simulink subsystem "thermal_model_stage_2"  (R2023a)
settings: Solver=VariableStepAuto  StartTime=0.0  StopTime=10.0  RelTol=1e-3
undefined symbols (not defined in the file or in its folder): coolant_initial_pressure, coolant_initial_temperature, coolant_tube_D, tcp_port_diameter, tcp_time_constant, tcv_orifice_diameter, tcv_time_constant
libraries: fl_lib x24, nesl_utility x21, SimscapeFluids_lib x4
settings Model: Creator=stefan.notter  LastModifiedBy=stefan.notter
settings OptimizationCC: ReuseModelBlockBuffer=off

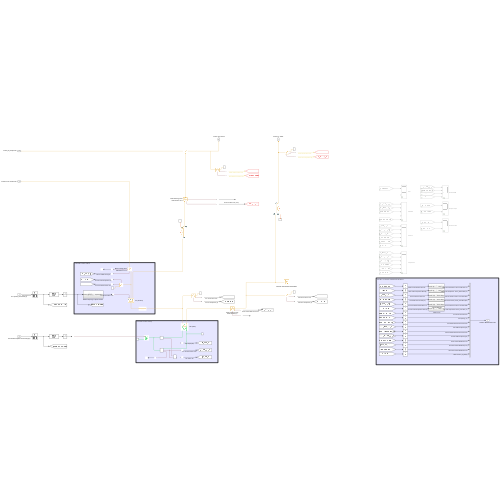
[thumbnail: Simulink's stored preview of the top-level diagram]
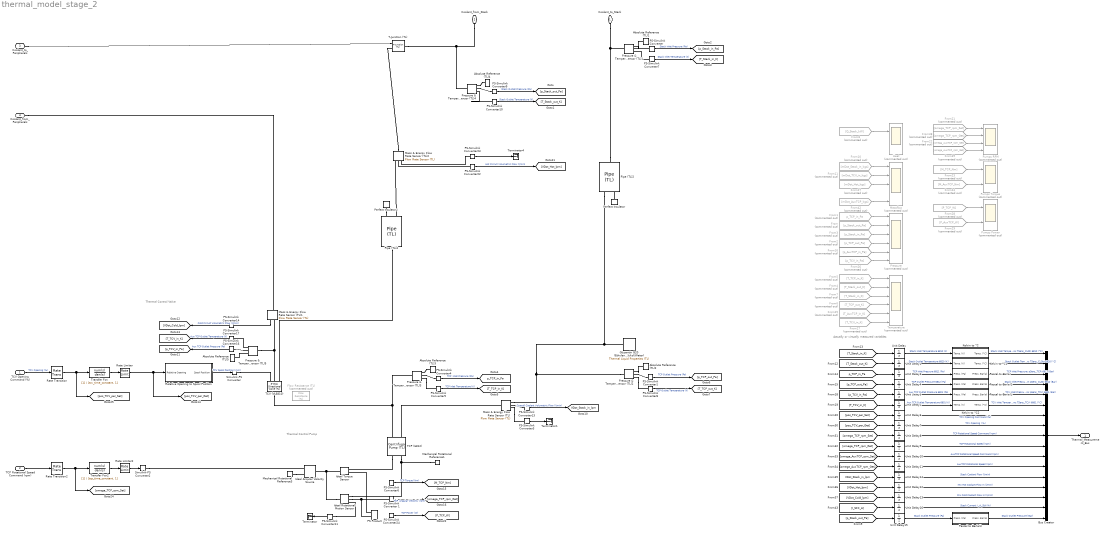
== system thermal_model_stage_2 ==
  note: Thermal Control Valve
  note: Actually or virtually measured variables
  note: Thermal Control Pump
  TCV Opening Command (%) : Inport
  TCP Rotational Speed Command (rpm) : Inport  Port=2
  Absolute Reference (TL){1..5} (5 alike) : fl_lib/Thermal Liquid/Elements/Absolute Reference (TL)
  Bus Creator : BusCreator  Inputs=17
  Flow Resistance (TL) : fl_lib/Thermal Liquid/Elements/Flow Resistance (TL)  Commented=on  delta_p_nominal=0.05 bar  mdot_nominal=1 kg/s  area=pi*tcv_orifice_diameter^2/4 m^2  laminar_fraction=1e-3
  From : From  Commented=on  GotoTag=p_Stack_out_Pa
  From1 : From  Commented=on  GotoTag=p_TCP_in_Pa  TagVisibility=global
  From10 : From  Commented=on  GotoTag=mDot_Stack_in_kgs  TagVisibility=global
  From11 : From  Commented=on  GotoTag=mDot_TCV_in_kgs
  From16 : From  Commented=on  GotoTag=p_AuxTCP_in_Pa
  From17 : From  Commented=on  GotoTag=T_TCV_in_K
  From2 : From  Commented=on  GotoTag=p_TCP_out_Pa
  From21 : From  Commented=on  GotoTag=omega_TCP_rpm_Set
  From22 : From  Commented=on  GotoTag=omega_AuxTCP_rpm_Set
  From23 : From  Commented=on  GotoTag=M_TCP_Nm
  From24 : From  Commented=on  GotoTag=M_AuxTCP_Nm
  From25 : From  Commented=on  GotoTag=T_AuxTCP_in_K
  From26 : From  Commented=on  GotoTag=p_TCV_in_Pa
  From27 : From  Commented=on  GotoTag=mDot_Hot_kgs
  From28 : From  Commented=on  GotoTag=P_TCP_W
  From29 : From  Commented=on  GotoTag=P_AuxTCP_W
  From3 : From  Commented=on  GotoTag=p_Stack_in_Pa
  From38 : From  Commented=on  GotoTag=omega_TCP_rpm_Get
  From39 : From  Commented=on  GotoTag=omega_AuxTCP_rpm_Get
  From4 : From  Commented=on  GotoTag=T_Stack_out_K
  From42 : From  Commented=on  GotoTag=mDot_AuxTCP_kgs
  From5 : From  Commented=on  GotoTag=T_TCP_in_K
  From6 : From  Commented=on  GotoTag=T_TCP_out_K
  From7 : From  Commented=on  GotoTag=T_Stack_in_K
  From8 : From  Commented=on  GotoTag=Q_Stack_kW  TagVisibility=global
  Glysantin G20 (Ethylenglykol/Water) : SimscapeFluids_lib/Thermal Liquid/Utilities/Thermal Liquid Properties (TL)  fluid_list=fluids.thermal_liquid.utilities.enum.thermal_liquid_fluid_list.ethylene_glycol  concentration_param_EG=fluids.thermal_liquid.utilities.enum.thermal_liquid_concentration.volume_fraction  concentration_param_PG=fluids.thermal_liquid.utilities.enum.thermal_liquid_concentration.volume_fraction  c_mass_SW=3.5e-3  c_mass_EG=0.1  c_mass_PG=0.1  c_mass_GL=0.1  c_vol_EG=0.5  c_vol_PG=0.1  beta_const_EG=2.1791 GPa  beta_const_PG=2.1791 GPa  beta_const_GL=2.1791 GPa  p_min_EG=0.01 MPa  p_min_PG=0.01 MPa  p_min_GL=0.01 MPa  p_max_EG=50 MPa  p_max_PG=50 MPa  p_max_GL=50 MPa  p_atm=coolant_initial_pressure MPa  properties_range_check=simscape.enum.assert.action.error
  Heat : Scope  Commented=on  NumInputPorts=2
  Ideal Angular Velocity Source : fl_lib/Mechanical/Mechanical Sources/Ideal Angular Velocity Source
  Ideal Rotational Motion Sensor : fl_lib/Mechanical/Mechanical Sensors/Ideal Rotational Motion Sensor  reference=foundation.enum.MeasurementReference.difference  acceleration_port=false  velocity_port=true  position_port=true  wrap_angle=false  offset=0 rad
  Ideal Torque Sensor : fl_lib/Mechanical/Mechanical Sensors/Ideal Torque Sensor
  Kelvin to °C : Subsystem
  Kelvin to °C1 : Subsystem
  Kelvin to °C2 : Subsystem
  Mass & Energy Flow Rate Sensor (TL) : fl_lib/Thermal Liquid/Sensors/Flow Rate Sensor (TL)  mass_flow_measure=false  volumetric_flow_measure=true  energy_flow_measure=true
      settings: InternalSimscapePortConfiguration="{\"Bottom\":[{\"id\":\"PHI\",\"label\":\"φ\",\"type\":\"output\"}],\"Left\":[{\"id\":\"A\",\"label\":\"A\",\"type\":\"foundation.thermal_liquid.thermal_liquid\"}],\"Right\":[{\"id\":\"B\",\"label\":\"B\",\"type\":\"foundation.thermal_liquid.thermal_liquid\"},{\"id\":\"V\",\"label\":\"V\",\"type\":\"output\"}],\"Top\":[]}"
  Mass & Energy Flow Rate Sensor (TL)1 : fl_lib/Thermal Liquid/Sensors/Flow Rate Sensor (TL)  mass_flow_measure=false  volumetric_flow_measure=true  energy_flow_measure=false
      settings: InternalSimscapePortConfiguration="{\"Bottom\":[],\"Left\":[{\"id\":\"A\",\"label\":\"A\",\"type\":\"foundation.thermal_liquid.thermal_liquid\"}],\"Right\":[{\"id\":\"B\",\"label\":\"B\",\"type\":\"foundation.thermal_liquid.thermal_liquid\"},{\"id\":\"V\",\"label\":\"V\",\"type\":\"output\"}],\"Top\":[]}"
  Mass & Energy Flow Rate Sensor (TL)2 : fl_lib/Thermal Liquid/Sensors/Flow Rate Sensor (TL)  mass_flow_measure=false  volumetric_flow_measure=true  energy_flow_measure=true
      settings: InternalSimscapePortConfiguration="{\"Bottom\":[{\"id\":\"PHI\",\"label\":\"φ\",\"type\":\"output\"}],\"Left\":[{\"id\":\"A\",\"label\":\"A\",\"type\":\"foundation.thermal_liquid.thermal_liquid\"}],\"Right\":[{\"id\":\"B\",\"label\":\"B\",\"type\":\"foundation.thermal_liquid.thermal_liquid\"},{\"id\":\"V\",\"label\":\"V\",\"type\":\"output\"}],\"Top\":[]}"
  Massflow : Scope  Commented=on  NumInputPorts=5
  Mechanical Rotational Reference1 : fl_lib/Mechanical/Rotational Elements/Mechanical Rotational Reference
  Mechanical Rotational Reference3 : fl_lib/Mechanical/Rotational Elements/Mechanical Rotational Reference
  PS Product : fl_lib/Physical Signals/Functions/PS Product
  PS-Simulink Converter{,1,3..5,7..11,16..17,23} (13 alike) : nesl_utility/PS-Simulink Converter  PhysicalDomain=network_engine_domain  SubClassName=ps_output  LeftPortType=input  RightPortType=output  PseudoPeriodic=off  Frequencies=[]  VectorFormat=inherit  Unit=inherit  AffineConversion=off
  PS-Simulink Converter 1 : nesl_utility/PS-Simulink Converter  PhysicalDomain=network_engine_domain  SubClassName=ps_output  LeftPortType=input  RightPortType=output  PseudoPeriodic=off  Frequencies=[]  VectorFormat=1-D array  Unit=rpm  AffineConversion=off
  PS-Simulink Converter13 : nesl_utility/PS-Simulink Converter  PhysicalDomain=network_engine_domain  SubClassName=ps_output  LeftPortType=input  RightPortType=output  PseudoPeriodic=off  Frequencies=[]  VectorFormat=inherit  Unit=l/min  AffineConversion=off
  PS-Simulink Converter14 : nesl_utility/PS-Simulink Converter  PhysicalDomain=network_engine_domain  SubClassName=ps_output  LeftPortType=input  RightPortType=output  PseudoPeriodic=off  Frequencies=[]  VectorFormat=inherit  Unit=l/min  AffineConversion=off
  PS-Simulink Converter22 : nesl_utility/PS-Simulink Converter  PhysicalDomain=network_engine_domain  SubClassName=ps_output  LeftPortType=input  RightPortType=output  PseudoPeriodic=off  Frequencies=[]  VectorFormat=inherit  Unit=l/min  AffineConversion=off
  PS-Simulink Converter24 : nesl_utility/PS-Simulink Converter  PhysicalDomain=network_engine_domain  SubClassName=ps_output  LeftPortType=input  RightPortType=output  PseudoPeriodic=off  Frequencies=[]  VectorFormat=inherit  Unit=W  AffineConversion=off
  PS-Simulink Converter6 : nesl_utility/PS-Simulink Converter  PhysicalDomain=network_engine_domain  SubClassName=ps_output  LeftPortType=input  RightPortType=output  PseudoPeriodic=off  Frequencies=[]  VectorFormat=inherit  Unit=N*m  AffineConversion=off
  Pascal to Bar(a) : Subsystem
  Pascal to Bar(a)1 : Subsystem
  Pascal to Bar(a)2 : Subsystem
  Pascal to Bar(a)3 : Subsystem
  Perfect Insulator : fl_lib/Thermal/Thermal Elements/Perfect Insulator  T_specify=off  T_priority=None  T=293.15 K  T_nominal_specify=off  T_nominal_unit=K  T_nominal_value=1
  Perfect Insulator2 : fl_lib/Thermal/Thermal Elements/Perfect Insulator  T_specify=off  T_priority=None  T=293.15 K  T_nominal_specify=off  T_nominal_unit=K  T_nominal_value=1
  Pipe (TL)2 : fl_lib/Thermal Liquid/Elements/Pipe (TL)  length=0.5 m  area=pi*coolant_tube_D^2/4 m^2  Dh=pi*coolant_tube_D*0.9 m  length_add=1 m  roughness=15e-6 m  Re_lam=2000  Re_tur=4000  shape_factor=64  Nu_lam=3.66  dynamic_compressibility=simscape.enum.onoff.on  inertia=simscape.enum.onoff.off  p0=coolant_initial_pressure MPa  T0=coolant_initial_temperature K  mdot0=0 kg/s
  Pipe (TL)4 : fl_lib/Thermal Liquid/Elements/Pipe (TL)  length=0.5 m  area=pi*coolant_tube_D^2/4 m^2  Dh=pi*coolant_tube_D*0.9 m  length_add=1 m  roughness=15e-6 m  Re_lam=2000  Re_tur=4000  shape_factor=64  Nu_lam=3.66  dynamic_compressibility=simscape.enum.onoff.on  inertia=simscape.enum.onoff.off  p0=coolant_initial_pressure MPa  T0=coolant_initial_temperature K  mdot0=0 kg/s
  Pressure : Scope  Commented=on  NumInputPorts=6
  Pressure & Temperature Sensor (TL){1..5} (5 alike) : fl_lib/Thermal Liquid/Sensors/Pressure & Temperature Sensor (TL)  reference=foundation.enum.MeasurementReference.difference  pressure=true  pressure_spec=foundation.enum.PressureMeasementSpec.Absolute  temperature=true
      settings: InternalSimscapePortConfiguration="{\"Bottom\":[{\"id\":\"T\",\"label\":\"T\",\"type\":\"output\"}],\"Left\":[{\"id\":\"A\",\"label\":\"A\",\"type\":\"foundation.thermal_liquid.thermal_liquid\"}],\"Right\":[{\"id\":\"B\",\"label\":\"B\",\"type\":\"foundation.thermal_liquid.thermal_liquid\"},{\"id\":\"P\",\"label\":\"P\",\"type\":\"output\"}],\"Top\":[]}"
  Pumps Power : Scope  Commented=on  NumInputPorts=2
  Pumps RPM : Scope  Commented=on  NumInputPorts=4
  Pumps Torque : Scope  Commented=on  NumInputPorts=2
  Rate Limiter : RateLimiter  RisingSlewLimit=45  FallingSlewLimit=-45  SampleTimeMode=inherited
  Rate Limiter2 : RateLimiter  RisingSlewLimit=1000  FallingSlewLimit=-1000  SampleTimeMode=inherited
  Rate Transition : RateTransition
  Rate Transition2 : RateTransition
  Relative Opening to Spool Position : Subsystem
  Simulink-PS Converter : nesl_utility/Simulink-PS Converter  PhysicalDomain=network_engine_domain  SubClassName=ps_input  LeftPortType=input  RightPortType=output  PseudoPeriodic=off  Frequencies=[]  NoiseDistribution=none  NoiseParameters=[]  Unit=mm  AffineConversion=off  FilteringAndDerivatives=provide  SimscapeFilterOrder=1  InputFilterTimeConstant=0.001  UdotUserProvided=0
  Simulink-PS Converter2 : nesl_utility/Simulink-PS Converter  PhysicalDomain=network_engine_domain  SubClassName=ps_input  LeftPortType=input  RightPortType=output  PseudoPeriodic=off  Frequencies=[]  NoiseDistribution=none  NoiseParameters=[]  Unit=rpm  AffineConversion=off  FilteringAndDerivatives=provide  SimscapeFilterOrder=1  InputFilterTimeConstant=0.001  UdotUserProvided=0
  T-Junction (TL) : SimscapeFluids_lib/Thermal Liquid/Pipes & Fittings/T-Junction (TL)  area_main=pi*coolant_tube_D^2/4 m^2  area_branch=pi*coolant_tube_D^2/4 m^2  junction_spec=fluids.thermal_liquid.pipes_fittings.enum.TLossCoefficientModel.Crane  k_main_converge=1.12  k_main_diverge=1.12  k_branch_converge=1.12  k_branch_diverge=1.12  radius=0.001 m  Re_c=150  saturation_ratio=0.2  mdot_A_specify=off  mdot_A_priority=High  mdot_A=0 kg/s  mdot_A_nominal_specify=off  mdot_A_nominal_unit=kg/s  mdot_A_nominal_value=1  mdot_B_specify=off  mdot_B_priority=High  mdot_B=0 kg/s  mdot_B_nominal_specify=off  mdot_B_nominal_unit=kg/s  mdot_B_nominal_value=1  mdot_C_specify=off  mdot_C_priority=High  mdot_C=0 kg/s  mdot_C_nominal_specify=off  mdot_C_nominal_unit=kg/s  mdot_C_nominal_value=1
      settings: InternalSimscapePortConfiguration="{\"Bottom\":[{\"id\":\"C\",\"label\":\"C\",\"type\":\"foundation.thermal_liquid.thermal_liquid\"}],\"Left\":[{\"id\":\"A\",\"label\":\"A\",\"type\":\"foundation.thermal_liquid.thermal_liquid\"}],\"Right\":[{\"id\":\"B\",\"label\":\"B\",\"type\":\"foundation.thermal_liquid.thermal_liquid\"}],\"Top\":[]}"
  TCP (6812) : SimscapeFluids_lib/Thermal Liquid/Pumps & Motors/Centrifugal Pump (TL)  pump_parameterization=fluids.thermal_liquid.pumps_motors.enum.CentrifugalPumpParameterization.Table2D  capacity_ref_nominal=6000/60 lpm  head_ref_nominal=|  power_ref_nominal=0.3 kW  head_ref_max=|  capacity_ref_max=12000/60 lpm  omega_ref_analytic=3500 rpm  flow_rate_1D_TLU=[1000, 2000, 3000, 4000, 5000, 6000, 7000, 8000, 9000, 1000] lpm  head_1D_TLU=[50, 47.5, 45, 40, 35, 25] m  power_1D_TLU=[.6, .75, .85, .93, .98, .99] kW  omega_ref_1D=3500 rpm  rho_ref_1D=998.21 kg/m^3  omega_threshold_factor=1e-2  flow_rate_2D_TLU=tcp_capacity_vector_lpm lpm  omega_2D_TLU=tcp_shaft_speed_vector_rpm rpm  head_2D_TLU=tcp_head_table_m m  power_2D_TLU=tcp_brake_power_table_kW kW  rho_ref_2D=tcp_reference_density kg/m^3  diameter_ratio=1  mech_orientation=fluids.thermal_liquid.pumps_motors.enum.CentrifugalPumpMechOrientation.Positive  area=pi/4*tcp_port_diameter^2 m^2
      head_ref_nominal=|
      | 1.2*10^5/(1000*9.81)
      |  m
      head_ref_max=|
      | 1.55*10^5/(1000*9.81)
      |  m
      settings: InternalSimscapePortConfiguration="{\"Bottom\":[],\"Left\":[{\"id\":\"A\",\"label\":\"A\",\"type\":\"foundation.thermal_liquid.thermal_liquid\"},{\"id\":\"B\",\"label\":\"B\",\"type\":\"foundation.thermal_liquid.thermal_liquid\"}],\"Right\":[{\"id\":\"R\",\"label\":\"R\",\"type\":\"foundation.mechanical.rotational.rotational\"},{\"id\":\"C\",\"label\":\"C\",\"type\":\"foundation.mechanical.rotational.rotational\"}],\"Top\":[]}"
  TCV (VL6810) : SimscapeFluids_lib/Thermal Liquid/Valves & Orifices/Directional Control Valves/3-Way Directional Valve (TL)  open_orifices_pos=fluids.thermal_liquid.valves.directional_control_valves.enum.OpenOrifices3Way.PA  open_orifices_neg=fluids.thermal_liquid.valves.directional_control_valves.enum.OpenOrifices3Way.AT  area_spec=fluids.thermal_liquid.valves.directional_control_valves.enum.area_spec.identical  valve_spec=fluids.thermal_liquid.valves.directional_control_valves.enum.ValveSpec.Table1DAreaOpening  del_S_max=5e-3 m  area_max=pi*tcv_orifice_diameter^2/4 m^2  del_S_TLU=tcv_spool_travel_vec m  valve_area_TLU=tcv_orifice_area_vec m^2  del_S_flow_TLU=[0, .002, .004, .007, .017] m  p_diff_TLU=[.3, .5, .7] bar  vol_flow_TLU=1e-3 * [1.7e-05, 2e-05, 2.6e-05; .0035, .0045, .0053; .7, .9, 1.06; 1.96, 2.5, 3; 6, 7.7, 9.13] lpm  mdot_TLU=[1.7e-05, 2e-05, 2.6e-05; .0035, .0045, .0053; .7, .9, 1.06; 1.96, 2.5, 3; 6, 7.7, 9.13] kg/s  T_ref_in=293.15 K  p_ref_in=0.101325 MPa  area_leak=tcv_leakage_area m^2  Cd=0.7  Re_c=12  smoothing_factor=0.01  pressure_recovery=simscape.enum.onoff.off  area=pi*coolant_tube_D^2/4 m^2  S_max_PA=2.5e-3 m  del_S_max_PA=0.005 m  area_max_PA=1e-4 m^2  del_S_TLU_PA=[0, .002, .004, .007, .017] m  valve_area_TLU_PA=[1e-09, 2.0352e-07, 4.0736e-05, .00011438, .00034356] m^2  del_S_flow_TLU_PA=[0, .002, .004, .007, .017] m  p_diff_TLU_PA=[.3, .5, .7] MPa  vol_flow_TLU_PA=1e-3 * [1.7e-05, 2e-05, 2.6e-05; .0035, .0045, .0053; .7, .9, 1.06; 1.96, 2.5, 3; 6, 7.7, 9.13] m^3/s  mdot_TLU_PA=[1.7e-05, 2e-05, 2.6e-05; .0035, .0045, .0053; .7, .9, 1.06; 1.96, 2.5, 3; 6, 7.7, 9.13] kg/s  S_max_AT=-2.5e-3 m  del_S_max_AT=0.005 m  area_max_AT=1e-4 m^2  del_S_TLU_AT=[0, .002, .004, .007, .017] m  valve_area_TLU_AT=[1e-09, 2.0352e-07, 4.0736e-05, .00011438, .00034356] m^2  del_S_flow_TLU_AT=[0, .002, .004, .007, .017] m  p_diff_TLU_AT=[.3, .5, .7] MPa  vol_flow_TLU_AT=1e-3 * [1.7e-05, 2e-05, 2.6e-05; .0035, .0045, .0053; .7, .9, 1.06; 1.96, 2.5, 3; 6, 7.7, 9.13] m^3/s  mdot_TLU_AT=[1.7e-05, 2e-05, 2.6e-05; .0035, .0045, .0053; .7, .9, 1.06; 1.96, 2.5, 3; 6, 7.7, 9.13] kg/s  S_max_PT=2.5e-3 m  del_S_max_PT=0.005 m  area_max_PT=1e-4 m^2  del_S_TLU_PT=[0, .002, .004, .007, .017] m  valve_area_TLU_PT=[1e-09, 2.0352e-07, 4.0736e-05, .00011438, .00034356] m^2  del_S_flow_TLU_PT=[0, .002, .004, .007, .017] m  p_diff_TLU_PT=[.3, .5, .7] MPa  vol_flow_TLU_PT=1e-3 * [1.7e-05, 2e-05, 2.6e-05; .0035, .0045, .0053; .7, .9, 1.06; 1.96, 2.5, 3; 6, 7.7, 9.13] m^3/s  mdot_TLU_PT=[1.7e-05, 2e-05, 2.6e-05; .0035, .0045, .0053; .7, .9, 1.06; 1.96, 2.5, 3; 6, 7.7, 9.13] kg/s
      settings: InternalSimscapePortConfiguration="{\"Bottom\":[],\"Left\":[{\"id\":\"A\",\"label\":\"A\",\"type\":\"foundation.thermal_liquid.thermal_liquid\"}],\"Right\":[{\"id\":\"S\",\"label\":\"S\",\"type\":\"input\"},{\"id\":\"P\",\"label\":\"P\",\"type\":\"foundation.thermal_liquid.thermal_liquid\"},{\"id\":\"T\",\"label\":\"T\",\"type\":\"foundation.thermal_liquid.thermal_liquid\"}],\"Top\":[]}"
  Temperature : Scope  Commented=on  NumInputPorts=6
  Terminator : Terminator
  Terminator1 : Terminator
  Terminator4 : Terminator
  Transfer Fcn : TransferFcn  Denominator=[tcv_time_constant, 1]  ContinuousStateAttributes='tcv_opening'
  Transfer Fcn2 : TransferFcn  Denominator=[tcp_time_constant, 1]  ContinuousStateAttributes='tcv_opening'
  Unit Delay : UnitDelay  InitialCondition=coolant_initial_temperature  SampleTime=-1  HasFrameUpgradeWarning=on
  Unit Delay1 : UnitDelay  InitialCondition=coolant_initial_temperature  SampleTime=-1  HasFrameUpgradeWarning=on
  Unit Delay{6..14,16} (10 alike) : UnitDelay  SampleTime=-1  HasFrameUpgradeWarning=on
  Unit Delay{3..5,15} (4 alike) : UnitDelay  InitialCondition=coolant_initial_pressure  SampleTime=-1  HasFrameUpgradeWarning=on
  Unit Delay2 : UnitDelay  InitialCondition=coolant_initial_temperature  SampleTime=-1  HasFrameUpgradeWarning=on
  Coolant_to_Stack : PMIOPort  Side=Left
  Coolant_from_Stack : PMIOPort  Port=2  Side=Left
  Coolant_to_Peripherals : PMIOPort  Port=3  Side=Right
  Coolant_from_Peripherals : PMIOPort  Port=4  Side=Right
  Thermal_Measurement_Bus : Outport
  tag scope: VDot_Stack_in_lpm=global, p_TCP_in_Pa=global
  wires:
  PS-Simulink Converter 1/1 -> [omega_TCP_rpm_Get]  "TCP  Angular Velocity (rpm)"
  Relative Opening to Spool Position/1(Spool Position) -> Simulink-PS Converter/1  "TCV Spool Position (mm)"
  PS-Simulink Converter11/1 -> Terminator/1
  PS-Simulink Converter6/1 -> [M_TCP_Nm]  "TCP Torque (Nm)"
  Bus Creator/1 -> Thermal_Measurement_Bus/1
  PS-Simulink Converter9/1 -> [p_Stack_out_Pa]  "Stack Outlet Pressure (Pa)"
  PS-Simulink Converter10/1 -> [T_Stack_out_K]  "Stack Outlet Temperature (K)"
  PS-Simulink Converter/1 -> [p_Stack_in_Pa]  "Stack Inlet Pressure (Pa)"
  PS-Simulink Converter7/1 -> [T_Stack_in_K]  "Stack Inlet Temperature (K)"
  PS-Simulink Converter5/1 -> [T_TCP_in_K]  "TCP Inlet Temperature (K)"
  PS-Simulink Converter4/1 -> [p_TCP_in_Pa]  "TCP  Inlet Pressure (Pa)"
  PS-Simulink Converter1/1 -> [p_TCP_out_Pa]  "TCP Outlet Pressure (Pa)"
  PS-Simulink Converter8/1 -> [T_TCP_out_K]  "TCP Outlet Temperature (K)"
  From2/1 -> Pressure/4
  From3/1 -> Pressure/3
  From/1 -> Pressure/2
  From1/1 -> Pressure/1
  From7/1 -> Temperature/3
  From6/1 -> Temperature/4
  From5/1 -> Temperature/1
  From4/1 -> Temperature/2
  From8/1 -> Heat/1
  PS-Simulink Converter3/1 -> Terminator1/1
  PS-Simulink Converter13/1 -> [VDot_Stack_in_lpm]  "Overall Coolant Volumetric Flow (l/min)"
  PS-Simulink Converter14/1 -> [VDot_Cold_lpm]  "Cold Circuit Volumetric Flow (l/min)"
  From10/1 -> Massflow/1
  From11/1 -> Massflow/2
  [T_Stack_out_K] -> Unit Delay1/1
  [T_Stack_in_K] -> Unit Delay/1
  [p_TCP_in_Pa] -> Unit Delay3/1
  [p_TCP_out_Pa] -> Unit Delay4/1
  PS-Simulink Converter16/1 -> [p_TCV_in_Pa]  "Aux TCP Outlet Pressure (Pa)"
  PS-Simulink Converter17/1 -> [T_TCV_in_K]  "Aux TCP Outlet Temperature (K)"
  From16/1 -> Pressure/5
  From17/1 -> Temperature/6
  [p_TCV_in_Pa] -> Unit Delay5/1
  [T_TCV_in_K] -> Unit Delay2/1
  [pos_TCV_per_Set] -> Unit Delay6/1
  From21/1 -> Pumps RPM/1
  From23/1 -> Pumps Torque/1
  From24/1 -> Pumps Torque/2
  From25/1 -> Temperature/5
  From26/1 -> Pressure/6
  PS-Simulink Converter22/1 -> [VDot_Hot_lpm]  "Hot Circuit Volumetric Flow (l/min)"
  PS-Simulink Converter23/1 -> Terminator4/1
  From27/1 -> Massflow/3
  TCP Rotational Speed Command (rpm)/1 -> Rate Transition2/1
  PS-Simulink Converter24/1 -> [P_TCP_W]  "TCP Power (W)"
  From28/1 -> Pumps Power/1
  From29/1 -> Pumps Power/2
  Unit Delay/1 -> Kelvin to °C/1(Temp. (K))  "Stack Inlet Temperature 6812 (K)"
  Unit Delay1/1 -> Kelvin to °C1/1(Temp. (K))  "Stack Outlet Temperature 6820 (K)"
  Unit Delay2/1 -> Kelvin to °C2/1(Temp. (K))  "Aux TCP Outlet Temperature 6801 (K)"
  Unit Delay3/1 -> Pascal to Bar(a)/1(Press. (Pa))  "TCP Inlet Pressure 6811 (Pa)"
  Unit Delay4/1 -> Pascal to Bar(a)1/1(Press. (Pa))  "TCP Outlet Pressure 6812 (Pa)"
  Unit Delay5/1 -> Pascal to Bar(a)2/1(Press. (Pa))  "Aux TCP Outlet Pressure 6801 (Pa)"
  Unit Delay6/1 -> Bus Creator/7  "TCV Opening Command (%)"
  Rate Limiter/1 -> Relative Opening to Spool Position/1(Relative Opening), [pos_TCV_per_Get]
  Rate Limiter2/1 -> Simulink-PS Converter2/1
  TCV Opening Command (%)/1 -> Rate Transition/1  "TCV Opening (%)"
  [pos_TCV_per_Get] -> Unit Delay7/1
  Unit Delay7/1 -> Bus Creator/8  "TCV Opening  (%)"
  Unit Delay9/1 -> Bus Creator/10  "TCP Rotational Speed (rpm)"
  [omega_TCP_rpm_Get] -> Unit Delay9/1
  [omega_TCP_rpm_Set] -> Unit Delay8/1
  Unit Delay8/1 -> Bus Creator/9  "TCP Rotational Speed Command (rpm)"
  [omega_AuxTCP_rpm_Get] -> Unit Delay11/1
  [omega_AuxTCP_rpm_Set] -> Unit Delay10/1
  Unit Delay10/1 -> Bus Creator/11  "AuxTCP Rotational Speed Command (rpm)"
  Unit Delay11/1 -> Bus Creator/12  "AuxTCP Rotational Speed (rpm)"
  Kelvin to °C/1(Temp. (°C)) -> Bus Creator/1  "Stack Inlet Temperature: TSens_CLSti 6812 (°C)"
  Kelvin to °C1/1(Temp. (°C)) -> Bus Creator/2  "Stack Outlet Temperature: TSens_CLSto 6820 (°C)"
  Kelvin to °C2/1(Temp. (°C)) -> Bus Creator/6  "TCV Inlet Temperature: TSens_TCVi 6801 (°C)"
  Pascal to Bar(a)/1(Press. Bar(a)) -> Bus Creator/3  "TCP Inlet Pressure: pSens_TCPi 6811 (Bar)"
  Pascal to Bar(a)1/1(Press. Bar(a)) -> Bus Creator/4  "Stack Inlet Pressure: pSens_CLSti 6812 (Bar)"
  Pascal to Bar(a)2/1(Press. Bar(a)) -> Bus Creator/5  "TCV Inlet Pressure: pSens_TCVi 6801 (Bar)"
  Rate Transition/1 -> [pos_TCV_per_Set], Transfer Fcn/1
  Transfer Fcn/1 -> Rate Limiter/1
  Transfer Fcn2/1 -> Rate Limiter2/1
  Rate Transition2/1 -> Transfer Fcn2/1, [omega_TCP_rpm_Set]
  Unit Delay13/1 -> Bus Creator/15  "Mix Cold Coolant Flow In (l/min)"
  Unit Delay12/1 -> Bus Creator/14  "Mix Hot Coolant Flow In (l/min)"
  [VDot_Stack_in_lpm] -> Unit Delay14/1
  Unit Delay14/1 -> Bus Creator/13  "Stack Coolant Flow (l/min)"
  [VDot_Cold_lpm] -> Unit Delay13/1
  [VDot_Hot_lpm] -> Unit Delay12/1
  From39/1 -> Pumps RPM/4
  From38/1 -> Pumps RPM/2
  From22/1 -> Pumps RPM/3
  From42/1 -> Massflow/5
  [I_SFC_A] -> Unit Delay16/1
  Unit Delay16/1 -> Bus Creator/16  "Stack Current: I_A_StN (A)"
  Unit Delay15/1 -> Pascal to Bar(a)3/1(Press. (Pa))  "Stack Outlet Pressure (Pa)"
  [p_Stack_out_Pa] -> Unit Delay15/1
  Pascal to Bar(a)3/1(Press. Bar(a)) -> Bus Creator/17  "Stack Outlet Pressure (Bar)"
  connections:
  Ideal Rotational Motion Sensor/LConn1 -- Ideal Torque Sensor/LConn1 -- Ideal Angular Velocity Source/LConn1
  Mechanical Rotational Reference1/LConn1 -- TCP (6812)/RConn2 -- Ideal Rotational Motion Sensor/RConn1
  Mass & Energy Flow Rate Sensor (TL)1/RConn1 -- TCV (VL6810)/RConn2 -- Pressure & Temperature Sensor (TL)5/LConn1
  PS Product/LConn2 -- PS-Simulink Converter 1/LConn1 -- Ideal Rotational Motion Sensor/RConn2
  Coolant_from_Stack/RConn1 -- Pressure & Temperature Sensor (TL)4/LConn1 -- T-Junction (TL)/LConn1
  TCV (VL6810)/LConn1 -- TCP (6812)/LConn1 -- Pressure & Temperature Sensor (TL)3/LConn1
  Pressure & Temperature Sensor (TL)2/LConn1 -- Glysantin G20 (Ethylenglykol/Water)/RConn1 -- Pipe (TL)2/LConn1 -- Mass & Energy Flow Rate Sensor (TL)/RConn1
  Pipe (TL)2/RConn1 -- Pressure & Temperature Sensor (TL)1/LConn1 -- Coolant_to_Stack/RConn1
  PS Product/LConn1 -- Ideal Torque Sensor/RConn2
  T-Junction (TL)/RConn2 -- Mass & Energy Flow Rate Sensor (TL)2/LConn1
  Mechanical Rotational Reference3/LConn1 -- Ideal Angular Velocity Source/RConn2
  PS-Simulink Converter11/LConn1 -- Ideal Rotational Motion Sensor/RConn3
  Simulink-PS Converter/RConn1 -- TCV (VL6810)/RConn1
  TCP (6812)/RConn1 -- Ideal Torque Sensor/RConn1
  Simulink-PS Converter2/RConn1 -- Ideal Angular Velocity Source/RConn1
  Absolute Reference (TL)1/LConn1 -- Pressure & Temperature Sensor (TL)1/RConn1
  PS-Simulink Converter7/LConn1 -- Pressure & Temperature Sensor (TL)1/RConn3
  Pressure & Temperature Sensor (TL)1/RConn2 -- PS-Simulink Converter/LConn1
  Absolute Reference (TL)2/LConn1 -- Pressure & Temperature Sensor (TL)2/RConn1
  Absolute Reference (TL)3/LConn1 -- Pressure & Temperature Sensor (TL)3/RConn1
  Pressure & Temperature Sensor (TL)4/RConn1 -- Absolute Reference (TL)4/LConn1
  Pressure & Temperature Sensor (TL)4/RConn2 -- PS-Simulink Converter9/LConn1
  PS-Simulink Converter10/LConn1 -- Pressure & Temperature Sensor (TL)4/RConn3
  Pressure & Temperature Sensor (TL)3/RConn2 -- PS-Simulink Converter4/LConn1
  Pressure & Temperature Sensor (TL)3/RConn3 -- PS-Simulink Converter5/LConn1
  Pressure & Temperature Sensor (TL)2/RConn3 -- PS-Simulink Converter8/LConn1
  Pressure & Temperature Sensor (TL)2/RConn2 -- PS-Simulink Converter1/LConn1
  Mass & Energy Flow Rate Sensor (TL)/RConn3 -- PS-Simulink Converter3/LConn1
  Mass & Energy Flow Rate Sensor (TL)/RConn2 -- PS-Simulink Converter13/LConn1
  Mass & Energy Flow Rate Sensor (TL)1/RConn2 -- PS-Simulink Converter14/LConn1
  Pressure & Temperature Sensor (TL)5/RConn3 -- PS-Simulink Converter17/LConn1
  Absolute Reference (TL)5/LConn1 -- Pressure & Temperature Sensor (TL)5/RConn1
  Pressure & Temperature Sensor (TL)5/RConn2 -- PS-Simulink Converter16/LConn1
  PS-Simulink Converter22/LConn1 -- Mass & Energy Flow Rate Sensor (TL)2/RConn2
  PS-Simulink Converter23/LConn1 -- Mass & Energy Flow Rate Sensor (TL)2/RConn3
  TCP (6812)/LConn2 -- Mass & Energy Flow Rate Sensor (TL)/LConn1
  Perfect Insulator/LConn1 -- Pipe (TL)2/LConn2
  Coolant_to_Peripherals/RConn1 -- T-Junction (TL)/RConn1
  Perfect Insulator2/LConn1 -- Pipe (TL)4/LConn2
  Pipe (TL)4/LConn1 -- Mass & Energy Flow Rate Sensor (TL)2/RConn1
  Pipe (TL)4/RConn1 -- TCV (VL6810)/RConn3
  Coolant_from_Peripherals/RConn1 -- Mass & Energy Flow Rate Sensor (TL)1/LConn1

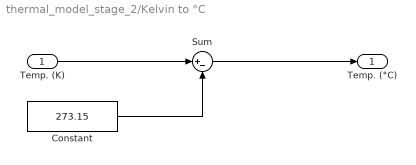
== system thermal_model_stage_2/Kelvin to °C ==
  Temp. (K) : Inport
  Constant : Constant  Value=273.15
  Sum : Sum  Inputs=|+-
  Temp. (°C) : Outport
  wires:
  Temp. (K)/1 -> Sum/1
  Sum/1 -> Temp. (°C)/1
  Constant/1 -> Sum/2

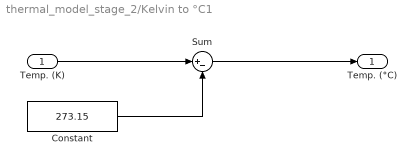
== system thermal_model_stage_2/Kelvin to °C1 ==
  Temp. (K) : Inport
  Constant : Constant  Value=273.15
  Sum : Sum  Inputs=|+-
  Temp. (°C) : Outport
  wires:
  Temp. (K)/1 -> Sum/1
  Sum/1 -> Temp. (°C)/1
  Constant/1 -> Sum/2

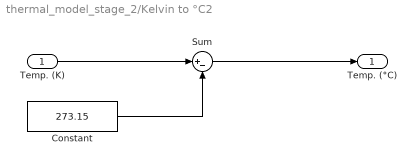
== system thermal_model_stage_2/Kelvin to °C2 ==
  Temp. (K) : Inport
  Constant : Constant  Value=273.15
  Sum : Sum  Inputs=|+-
  Temp. (°C) : Outport
  wires:
  Temp. (K)/1 -> Sum/1
  Sum/1 -> Temp. (°C)/1
  Constant/1 -> Sum/2

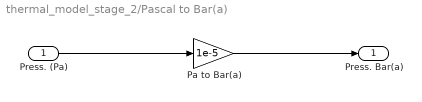
== system thermal_model_stage_2/Pascal to Bar(a) ==
  Press. (Pa) : Inport
  Pa to Bar(a) : Gain  Gain=1e-5
  Press. Bar(a) : Outport
  wires:
  Press. (Pa)/1 -> Pa to Bar(a)/1
  Pa to Bar(a)/1 -> Press. Bar(a)/1

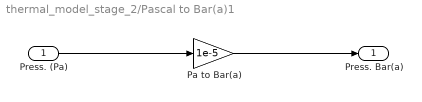
== system thermal_model_stage_2/Pascal to Bar(a)1 ==
  Press. (Pa) : Inport
  Pa to Bar(a) : Gain  Gain=1e-5
  Press. Bar(a) : Outport
  wires:
  Press. (Pa)/1 -> Pa to Bar(a)/1
  Pa to Bar(a)/1 -> Press. Bar(a)/1

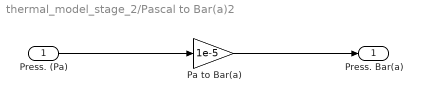
== system thermal_model_stage_2/Pascal to Bar(a)2 ==
  Press. (Pa) : Inport
  Pa to Bar(a) : Gain  Gain=1e-5
  Press. Bar(a) : Outport
  wires:
  Press. (Pa)/1 -> Pa to Bar(a)/1
  Pa to Bar(a)/1 -> Press. Bar(a)/1

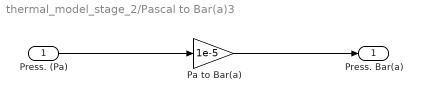
== system thermal_model_stage_2/Pascal to Bar(a)3 ==
  Press. (Pa) : Inport
  Pa to Bar(a) : Gain  Gain=1e-5
  Press. Bar(a) : Outport
  wires:
  Pa to Bar(a)/1 -> Press. Bar(a)/1
  Press. (Pa)/1 -> Pa to Bar(a)/1

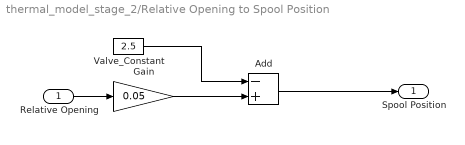
== system thermal_model_stage_2/Relative Opening to Spool Position ==
  Relative Opening : Inport
  Add : Sum  Inputs=-+
  Gain : Gain  Gain=0.05
  Valve_Constant : Constant  Value=2.5
  Spool Position : Outport
  wires:
  Add/1 -> Spool Position/1
  Valve_Constant/1 -> Add/1
  Relative Opening/1 -> Gain/1
  Gain/1 -> Add/2
